simulink model "iir"  (R2025b)
settings: Solver=FixedStepDiscrete  StartTime=0.0  StopTime=65  FixedStep=1  RelTol=1e-3
libraries: dspsrcs4 x1
settings Model: Creator=auralius  LastModifiedBy=auralius

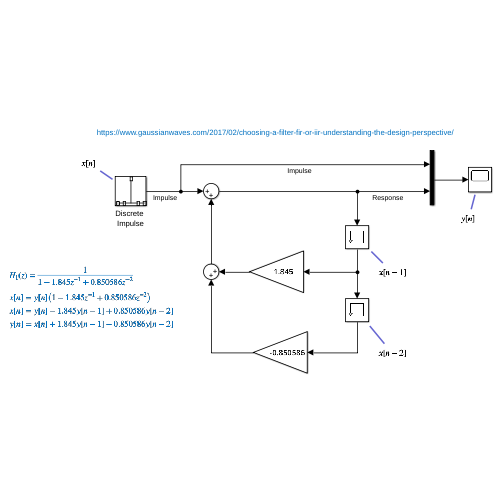
[thumbnail: Simulink's stored preview of the top-level diagram]
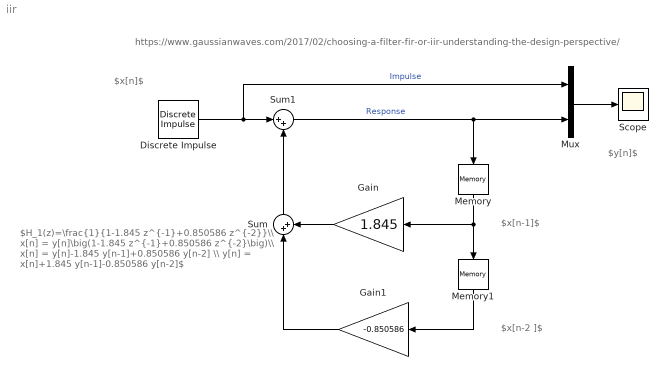
== system iir ==
  note: $x[n-1]$
  note: $y[n]$
  note: $x[n]$
  note: $H_1(z)=\frac{1}{1-1.845 z^{-1}+0.850586 z^{-2}}\\ x[n] = y[n]\big(1-1.845 z^{-1}+0.850586 z^{-2}\big)\\ x[n] = y[n]-1.845 y[n-1]+0.850586 y[n-2] \\ y[n] = x[n]+1.845 y[n-1]-0.850586 y[n-2]$
  note: https://www.gaussianwaves.com/2017/02/choosing-a-filter-fir-or-iir-understanding-the-design-perspective/
  note: $x[n-2 ]$
  Discrete Impulse : dspsrcs4/Discrete  Impulse  SFcnStateName=COUNT  Delay=0  SampleTime=1  FrameSample=1  OutputFrames=off  dataType=double  isSigned=on  wordLen=16  udDataType=sfix(16)  fracBitsMode=Best precision  numFracBits=15  OutDataTypeStr=double  LastOutDataTypeStr=double
      settings: SFcnIsStateOwnerBlock=on
  Gain : Gain  Gain=1.845
  Gain1 : Gain  Gain=-0.850586
  Memory : Memory
  Memory1 : Memory
  Mux : Mux  Inputs=2
  Scope : Scope
      settings: ActiveDisplayYMinimum=-0.62395469571180118  ActiveDisplayYMaximum=5.6155922614062117
  Sum : Sum  Inputs=|++
  Sum1 : Sum  Inputs=|++
  wires:
  Memory/1 -> Memory1/1, Gain/1
  Memory1/1 -> Gain1/1
  Gain1/1 -> Sum/1
  Gain/1 -> Sum/2
  Sum/1 -> Sum1/2
  Discrete Impulse/1 -> Mux/1, Sum1/1  "Impulse"
  Sum1/1 -> Mux/2, Memory/1  "Response"
  Mux/1 -> Scope/1
